simulink model "TuneNLMS"  (R2020b)
settings: Solver=VariableStepAuto  StartTime=0.0  StopTime=20  RelTol=1e-3
undefined symbols (not defined in the file): Controller_Mode, DiscIntNeverNeededParam, plant_N
libraries: dspadpt3 x5, dsparch4 x1, simulink x1
settings Model: DataDictionary=Dictionary.sldd  Creator=elbit  LastModifiedBy=elbit

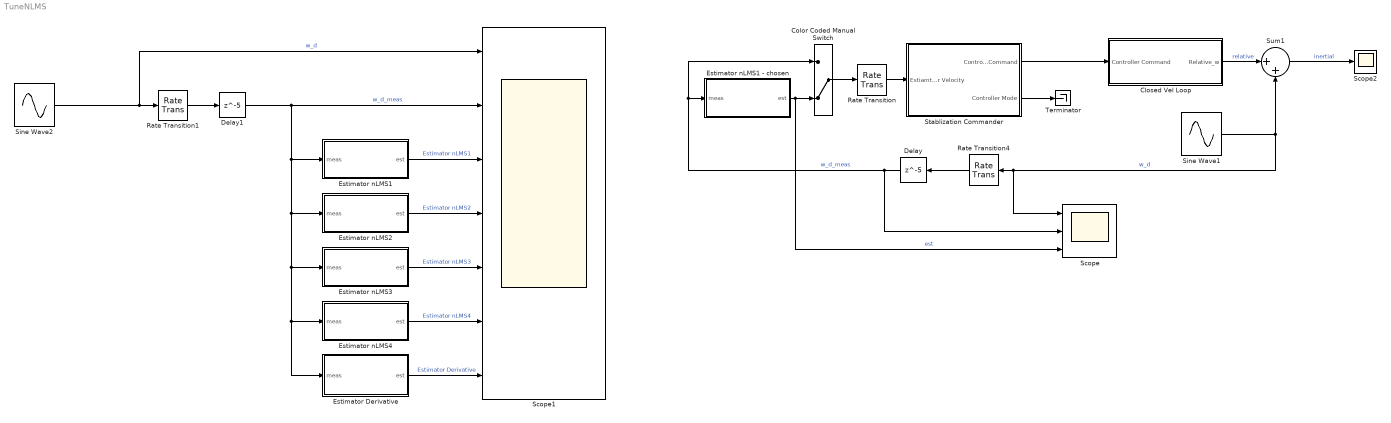
== system TuneNLMS ==
  Closed Vel Loop : Subsystem
  Color Coded Manual Switch : ManualSwitch  CurrentSetting=0
      settings: OpenFcn=|
      | sw = get_param(gcb,'sw');
      | if strcmp(sw,'1')
      | set_param(gcb,'sw','0');
      | else
      | set_param(gcb,'sw','1');
      | end
      | if strcmp(sw,'1')
      |     set_param(gcb,'backgroundcolor','red')
      | else
      |     set_param(gcb,'backgroundcolor','green')
      | end
  Delay : Delay  DelayLength=5
  Delay1 : Delay  DelayLength=5
  Estimator Derivative : Subsystem
  Estimator nLMS1 : Subsystem
  Estimator nLMS1 - chosen : Subsystem
  Estimator nLMS2 : Subsystem
  Estimator nLMS3 : Subsystem
  Estimator nLMS4 : Subsystem
  Rate Transition : RateTransition  OutPortSampleTime=ts_control
  Rate Transition1 : RateTransition  OutPortSampleTime=ts_camera
  Rate Transition4 : RateTransition  OutPortSampleTime=ts_camera
  Scope : Scope  NumInputPorts=3
  Scope1 : Scope  NumInputPorts=7
  Scope2 : Scope
  Sine Wave1 : Sin  Frequency=2*pi*1  SampleTime=0
  Sine Wave2 : Sin  Frequency=2*pi*1  SampleTime=0
  Stablization Commander : Subsystem  TreatAsAtomicUnit=on
  Sum1 : Sum  Inputs=|++
  Terminator : Terminator
  wires:
  Closed Vel Loop/1(Relative_w) -> Sum1/1  "relative"
  Sine Wave1/1 -> Scope/1, Rate Transition4/1, Sum1/2  "w_d"
  Stablization Commander/2(Controller Mode) -> Terminator/1
  Sum1/1 -> Scope2/1  "inertial"
  Rate Transition4/1 -> Delay/1
  Stablization Commander/1(Controller Command) -> Closed Vel Loop/1(Controller Command)
  Delay/1 -> Scope/2, Color Coded Manual Switch/1, Estimator nLMS1 - chosen/1(meas)  "w_d_meas"
  Rate Transition1/1 -> Delay1/1
  Sine Wave2/1 -> Scope1/1, Rate Transition1/1  "w_d"
  Delay1/1 -> Estimator nLMS2/1(meas), Estimator nLMS3/1(meas), Estimator nLMS4/1(meas), Estimator Derivative/1(meas), Estimator nLMS1/1(meas), Scope1/2  "w_d_meas"
  Estimator nLMS1/1(est) -> Scope1/3  "Estimator nLMS1"
  Estimator nLMS2/1(est) -> Scope1/4  "Estimator nLMS2"
  Color Coded Manual Switch/1 -> Rate Transition/1
  Estimator nLMS1 - chosen/1(est) -> Color Coded Manual Switch/2, Scope/3  "est"
  Rate Transition/1 -> Stablization Commander/1(Estiamted Base Angular Velocity)
  Estimator Derivative/1(est) -> Scope1/7  "Estimator Derivative"
  Estimator nLMS3/1(est) -> Scope1/5  "Estimator nLMS3"
  Estimator nLMS4/1(est) -> Scope1/6  "Estimator nLMS4"

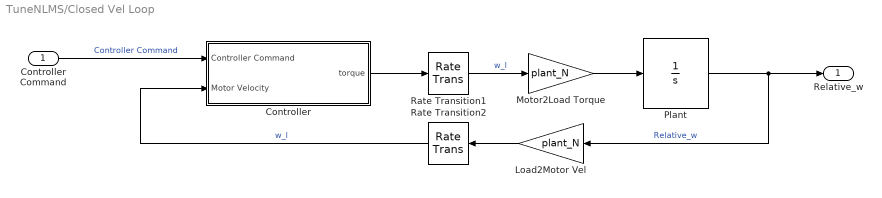
== system TuneNLMS/Closed Vel Loop ==
  Controller Command : Inport
  Controller : Subsystem
  Load2Motor Vel : Gain  Gain=plant_N
  Motor2Load Torque : Gain  Gain=plant_N
  Plant : Integrator
  Rate Transition1 : RateTransition  OutPortSampleTime=0
  Rate Transition2 : RateTransition  OutPortSampleTime=ts_control
  Relative_w : Outport
  wires:
  Controller Command/1 -> Controller/1(Controller Command)  "Controller Command"
  Controller/1(torque) -> Rate Transition1/1
  Plant/1 -> Load2Motor Vel/1, Relative_w/1  "Relative_w"
  Rate Transition2/1 -> Controller/2(Motor Velocity)  "w_l"
  Motor2Load Torque/1 -> Plant/1
  Rate Transition1/1 -> Motor2Load Torque/1  "w_l"
  Load2Motor Vel/1 -> Rate Transition2/1

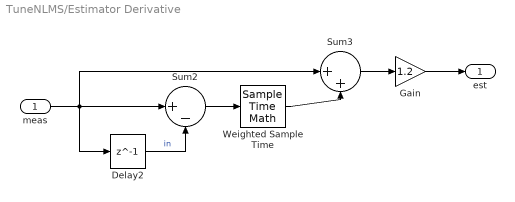
== system TuneNLMS/Estimator Derivative ==
  meas : Inport
  Delay2 : Delay  DelayLength=1
  Gain : Gain  Gain=1.2
  Sum2 : Sum  Inputs=|+-
  Sum3 : Sum  Inputs=|++
  Weighted Sample Time : SampleTimeMath  TsampMathOp=Ts Only
  est : Outport
  wires:
  Delay2/1 -> Sum2/2  "in"
  Sum2/1 -> Weighted Sample Time/1
  Weighted Sample Time/1 -> Sum3/2
  Sum3/1 -> Gain/1
  Gain/1 -> est/1
  meas/1 -> Delay2/1, Sum3/1, Sum2/1

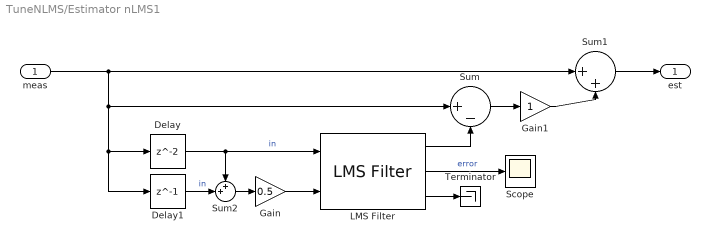
== system TuneNLMS/Estimator nLMS1 ==
  meas : Inport
  Delay : Delay
  Delay1 : Delay  DelayLength=1
  Gain : Gain  Gain=0.5
  Gain1 : Gain
  LMS Filter : dspadpt3/LMS Filter  Algo=Normalized LMS  L=9  stepflag=Dialog  mu=0.1  leakage=1  ic=0  Adapt=off  resetflag=None  weights=on  addnparflag=off  roundingMode=Floor  overflowMode=off  secondCoeffMode=Binary point scaling  secondCoeffWordLength=2  secondCoeffFracLength=15  prodOutput2Mode=Binary point scaling  prodOutput2FracLength=20  prodOutput3Mode=Binary point scaling  prodOutput3FracLength=20  prodOutput4Mode=Binary point scaling  prodOutput4FracLength=20  quotientMode=Binary point scaling  quotientFracLength=20  accum2Mode=Binary point scaling  accum2FracLength=20
      settings: SourceProductName=DSP System Toolbox
  Scope : Scope
  Sum : Sum  Inputs=|+-
  Sum1 : Sum  Inputs=|++
  Sum2 : Sum  Inputs=++|
  Terminator : Terminator
  est : Outport
  wires:
  LMS Filter/3 -> Terminator/1
  LMS Filter/2 -> Scope/1  "error"
  meas/1 -> Sum1/1, Sum/1, Delay1/1, Delay/1
  Delay/1 -> Sum2/1, LMS Filter/1  "in"
  LMS Filter/1 -> Sum/2
  Sum/1 -> Gain1/1
  Gain1/1 -> Sum1/2
  Sum1/1 -> est/1
  Delay1/1 -> Sum2/2  "in"
  Sum2/1 -> Gain/1
  Gain/1 -> LMS Filter/2

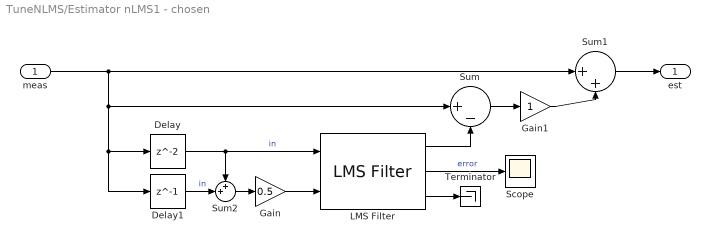
== system TuneNLMS/Estimator nLMS1 - chosen ==
  meas : Inport
  Delay : Delay
  Delay1 : Delay  DelayLength=1
  Gain : Gain  Gain=0.5
  Gain1 : Gain
  LMS Filter : dspadpt3/LMS Filter  Algo=Normalized LMS  L=9  stepflag=Dialog  mu=0.1  leakage=1  ic=0  Adapt=off  resetflag=None  weights=on  addnparflag=off  roundingMode=Floor  overflowMode=off  secondCoeffMode=Binary point scaling  secondCoeffWordLength=2  secondCoeffFracLength=15  prodOutput2Mode=Binary point scaling  prodOutput2FracLength=20  prodOutput3Mode=Binary point scaling  prodOutput3FracLength=20  prodOutput4Mode=Binary point scaling  prodOutput4FracLength=20  quotientMode=Binary point scaling  quotientFracLength=20  accum2Mode=Binary point scaling  accum2FracLength=20
      settings: SourceProductName=DSP System Toolbox
  Scope : Scope
  Sum : Sum  Inputs=|+-
  Sum1 : Sum  Inputs=|++
  Sum2 : Sum  Inputs=++|
  Terminator : Terminator
  est : Outport
  wires:
  LMS Filter/3 -> Terminator/1
  LMS Filter/2 -> Scope/1  "error"
  meas/1 -> Sum1/1, Sum/1, Delay1/1, Delay/1
  Delay/1 -> Sum2/1, LMS Filter/1  "in"
  LMS Filter/1 -> Sum/2
  Sum/1 -> Gain1/1
  Gain1/1 -> Sum1/2
  Sum1/1 -> est/1
  Delay1/1 -> Sum2/2  "in"
  Sum2/1 -> Gain/1
  Gain/1 -> LMS Filter/2

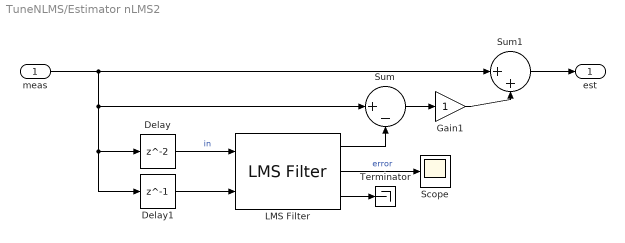
== system TuneNLMS/Estimator nLMS2 ==
  meas : Inport
  Delay : Delay
  Delay1 : Delay  DelayLength=1
  Gain1 : Gain
  LMS Filter : dspadpt3/LMS Filter  Algo=Normalized LMS  L=32  stepflag=Dialog  mu=0.1  leakage=1  ic=0  Adapt=off  resetflag=None  weights=on  addnparflag=off  roundingMode=Floor  overflowMode=off  secondCoeffMode=Binary point scaling  secondCoeffWordLength=2  secondCoeffFracLength=15  prodOutput2Mode=Binary point scaling  prodOutput2FracLength=20  prodOutput3Mode=Binary point scaling  prodOutput3FracLength=20  prodOutput4Mode=Binary point scaling  prodOutput4FracLength=20  quotientMode=Binary point scaling  quotientFracLength=20  accum2Mode=Binary point scaling  accum2FracLength=20
      settings: SourceProductName=DSP System Toolbox
  Scope : Scope
  Sum : Sum  Inputs=|+-
  Sum1 : Sum  Inputs=|++
  Terminator : Terminator
  est : Outport
  wires:
  LMS Filter/3 -> Terminator/1
  LMS Filter/2 -> Scope/1  "error"
  meas/1 -> Sum1/1, Sum/1, Delay1/1, Delay/1
  Delay/1 -> LMS Filter/1  "in"
  LMS Filter/1 -> Sum/2
  Sum/1 -> Gain1/1
  Gain1/1 -> Sum1/2
  Sum1/1 -> est/1
  Delay1/1 -> LMS Filter/2

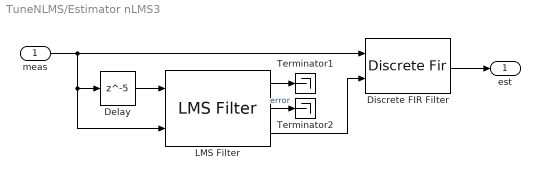
== system TuneNLMS/Estimator nLMS3 ==
  meas : Inport
  Delay : Delay  DelayLength=5
  Discrete FIR Filter : DiscreteFir  CoefSource=Input port  InputProcessing=Columns as channels (frame based)
      settings: InputPortMap=u0,u1
  LMS Filter : dspadpt3/LMS Filter  Algo=Normalized LMS  L=32  stepflag=Dialog  mu=0.1  leakage=1  ic=0  Adapt=off  resetflag=None  weights=on  addnparflag=off  roundingMode=Floor  overflowMode=off  secondCoeffMode=Binary point scaling  secondCoeffWordLength=2  secondCoeffFracLength=15  prodOutput2Mode=Binary point scaling  prodOutput2FracLength=20  prodOutput3Mode=Binary point scaling  prodOutput3FracLength=20  prodOutput4Mode=Binary point scaling  prodOutput4FracLength=20  quotientMode=Binary point scaling  quotientFracLength=20  accum2Mode=Binary point scaling  accum2FracLength=20
      settings: SourceProductName=DSP System Toolbox
  Terminator1 : Terminator
  Terminator2 : Terminator
  est : Outport
  wires:
  LMS Filter/1 -> Terminator1/1
  LMS Filter/3 -> Discrete FIR Filter/2
  meas/1 -> Delay/1, LMS Filter/2, Discrete FIR Filter/1
  LMS Filter/2 -> Terminator2/1  "error"
  Discrete FIR Filter/1 -> est/1
  Delay/1 -> LMS Filter/1

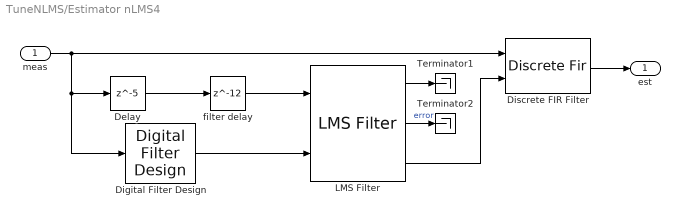
== system TuneNLMS/Estimator nLMS4 ==
  meas : Inport
  Delay : Delay  DelayLength=5
  Digital Filter Design : dsparch4/Digital Filter Design  mwdsp_browser_bugfix_var=off
  Discrete FIR Filter : DiscreteFir  CoefSource=Input port  InputProcessing=Columns as channels (frame based)
      settings: InputPortMap=u0,u1
  LMS Filter : dspadpt3/LMS Filter  Algo=Normalized LMS  L=32  stepflag=Dialog  mu=0.1  leakage=1  ic=0  Adapt=off  resetflag=None  weights=on  addnparflag=off  roundingMode=Floor  overflowMode=off  secondCoeffMode=Binary point scaling  secondCoeffWordLength=2  secondCoeffFracLength=15  prodOutput2Mode=Binary point scaling  prodOutput2FracLength=20  prodOutput3Mode=Binary point scaling  prodOutput3FracLength=20  prodOutput4Mode=Binary point scaling  prodOutput4FracLength=20  quotientMode=Binary point scaling  quotientFracLength=20  accum2Mode=Binary point scaling  accum2FracLength=20
      settings: SourceProductName=DSP System Toolbox
  Terminator1 : Terminator
  Terminator2 : Terminator
  filter delay : Delay  DelayLength=12
  est : Outport
  wires:
  LMS Filter/1 -> Terminator1/1
  LMS Filter/3 -> Discrete FIR Filter/2
  meas/1 -> Digital Filter Design/1, Delay/1, Discrete FIR Filter/1
  LMS Filter/2 -> Terminator2/1  "error"
  Discrete FIR Filter/1 -> est/1
  filter delay/1 -> LMS Filter/1
  Delay/1 -> filter delay/1
  Digital Filter Design/1 -> LMS Filter/2

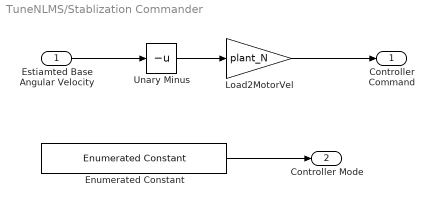
== system TuneNLMS/Stablization Commander ==
  Estiamted Base Angular Velocity : Inport
  Enumerated Constant : simulink/Sources/Enumerated Constant  OutDataTypeStr=Enum: Controller_Mode  Value=Controller_Mode.Velocity  SampleTime=inf
  Load2MotorVel : Gain  Gain=plant_N
  Unary Minus : UnaryMinus
  Controller Command : Outport
  Controller Mode : Outport  Port=2
  wires:
  Enumerated Constant/1 -> Controller Mode/1
  Estiamted Base Angular Velocity/1 -> Unary Minus/1
  Load2MotorVel/1 -> Controller Command/1
  Unary Minus/1 -> Load2MotorVel/1

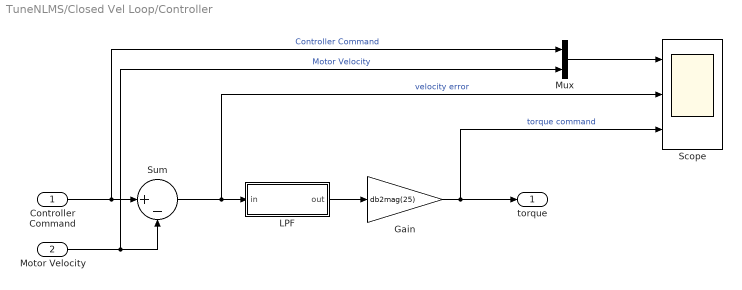
== system TuneNLMS/Closed Vel Loop/Controller ==
  Controller Command : Inport
  Motor Velocity : Inport  Port=2
  Gain : Gain  Gain=db2mag(25)
  LPF : Subsystem
  Mux : Mux  Inputs=2
  Scope : Scope  NumInputPorts=3
  Sum : Sum  Inputs=|+-
  torque : Outport
  wires:
  Gain/1 -> Scope/3, torque/1  "torque command"
  Controller Command/1 -> Mux/1, Sum/1  "Controller Command"
  Motor Velocity/1 -> Mux/2, Sum/2  "Motor Velocity"
  Mux/1 -> Scope/1
  LPF/1(out) -> Gain/1
  Sum/1 -> Scope/2, LPF/1(in)  "velocity error"

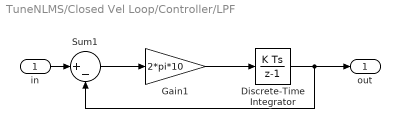
== system TuneNLMS/Closed Vel Loop/Controller/LPF ==
  in : Inport
  Discrete-Time Integrator : DiscreteIntegrator  SampleTime=-1  ICPrevOutput=DiscIntNeverNeededParam  ICPrevScaledInput=DiscIntNeverNeededParam
  Gain1 : Gain  Gain=2*pi*10
  Sum1 : Sum  Inputs=|+-
  out : Outport
  wires:
  Sum1/1 -> Gain1/1
  Discrete-Time Integrator/1 -> out/1, Sum1/2
  Gain1/1 -> Discrete-Time Integrator/1
  in/1 -> Sum1/1
